simulink model "Quadcopter_LQR_Discrete"  (R2016b)
settings: Solver=ode45  StartTime=0.0  StopTime=50  RelTol=1e-3  EnableMultiTasking=on
undefined symbols (not defined in the file): C, F, sigbuilder_block, Ts, X0
settings Model: Creator=Toshiba  LastModifiedBy=AAstudillo
settings DataIOCC: LimitDataPoints=on  SaveFormat=Array  SignalLoggingSaveFormat=ModelDataLogs
settings OptimizationCC: LifeSpan=inf
settings DebuggingCC: SolverPrmCheckMsg=warning  MultiTaskDSMMsg=warning  MultiTaskCondExecSysMsg=none  SFUnexpectedBacktrackingDiag=warning  SFNoUnconditionalDefaultTransitionDiag=warning  SFExecutionAtInitializationDiag=none
settings HardwareCC: ProdBitPerPointer=32  ProdBitPerSizeT=32  ProdBitPerPtrDiffT=32  ProdLargestAtomicFloat=None  ProdIntDivRoundTo=Undefined  ProdEndianess=Unspecified  ProdWordSize=32  ProdHWDeviceType=32-bit Generic
settings ModelReferenceCC: PropagateSignalLabelsOutOfModel=off
settings GRTTargetCC: TargetLangStandard=C89/C90 (ANSI)  GeneratePreprocessorConditionals=Disable all
settings ConfigComp: CovMetricSettings=dw  CovHtmlReporting=on  CovSaveCumulativeToWorkspaceVar=on  CovSaveSingleToWorkspaceVar=on  CovExternalEMLEnable=off

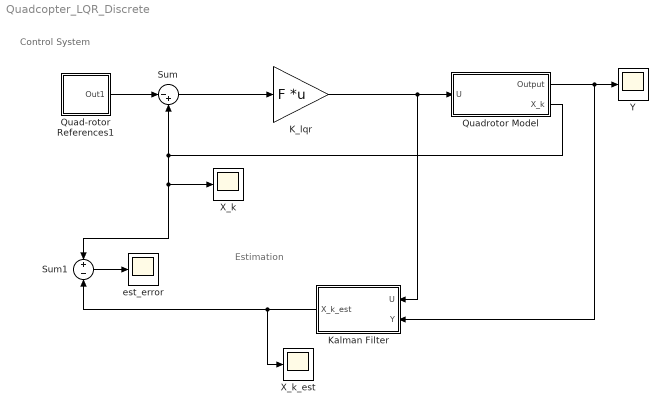
== system Quadcopter_LQR_Discrete ==
  note: Estimation
  note: Control System
  K_lqr : Gain  Gain=F  Multiplication=Matrix(K*u) (u vector)
  Kalman Filter : Subsystem
  Quad-rotor References1 : Subsystem
  Quadrotor Model : Subsystem
  Sum : Sum  Inputs=|-+
  Sum1 : Sum  Inputs=+|-
  X_k : Scope
  X_k_est : Scope
  Y : Scope
  est_error : Scope
  wires:
  K_lqr/1 -> Quadrotor Model/1(U), Kalman Filter/1(U)
  Sum/1 -> K_lqr/1
  Quadrotor Model/1("Output ") -> Y/1, Kalman Filter/2(Y)
  Quad-rotor References1/1(Out1) -> Sum/1
  Quadrotor Model/2(X_k) -> Sum1/1, X_k/1, Sum/2
  Kalman Filter/1("X_k_est ") -> X_k_est/1, Sum1/2
  Sum1/1 -> est_error/1

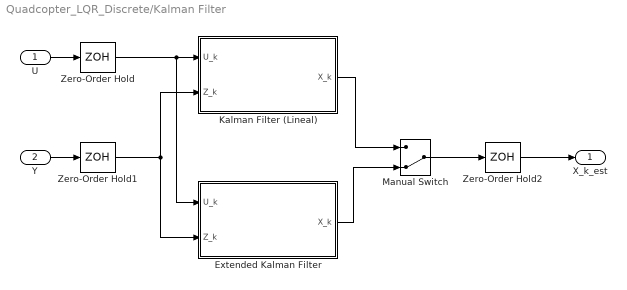
== system Quadcopter_LQR_Discrete/Kalman Filter ==
  U : Inport  PortDimensions=4
  Y : Inport  Port=2
  Extended Kalman Filter : MATLAB Function  TreatAsAtomicUnit=on
  Kalman Filter (Lineal) : MATLAB Function  TreatAsAtomicUnit=on
  Manual Switch : ManualSwitch  CurrentSetting=0
  Zero-Order Hold : ZeroOrderHold  SampleTime=Ts
  Zero-Order Hold1 : ZeroOrderHold  SampleTime=Ts
  Zero-Order Hold2 : ZeroOrderHold  SampleTime=Ts
  "X_k_est " : Outport  PortDimensions=12
  wires:
  U/1 -> Zero-Order Hold/1
  Zero-Order Hold/1 -> Extended Kalman Filter/1(U_k), Kalman Filter (Lineal)/1(U_k)
  Y/1 -> Zero-Order Hold1/1
  Zero-Order Hold1/1 -> Extended Kalman Filter/2(Z_k), Kalman Filter (Lineal)/2(Z_k)
  Kalman Filter (Lineal)/1(X_k) -> Manual Switch/1
  Zero-Order Hold2/1 -> "X_k_est "/1
  Extended Kalman Filter/1(X_k) -> Manual Switch/2
  Manual Switch/1 -> Zero-Order Hold2/1

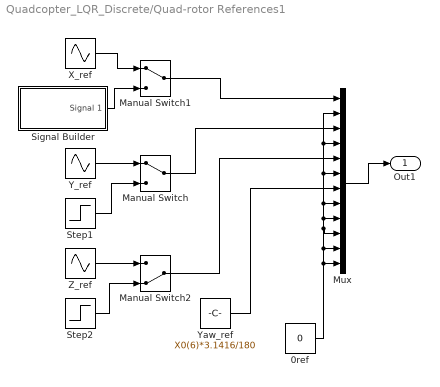
== system Quadcopter_LQR_Discrete/Quad-rotor References1 ==
  "0ref " : Constant  Value=0
  Manual Switch : ManualSwitch
  Manual Switch1 : ManualSwitch
  Manual Switch2 : ManualSwitch  CurrentSetting=0
  Mux : Mux  Inputs=12
  Signal Builder : Subsystem  Tag=STV Subsys  LoadFcn=sigbuilder_block('load');  StartFcn=sigbuilder_block('start');  StopFcn=sigbuilder_block('stop');  ClipboardFcn=sigbuilder_block('clipboard');  mask(Sigbuilder block){tuvar=[0:10]}
      mask help: Simulink:masks:SigbuilderBlock_MD
      mask init:
      | if ~strcmp(get_param(bdroot(gcbh),'SimulationStatus'),'stopped') tuvar = sigbuilder_block('maskInit'); end
      settings: CopyFcn=sigbuilder_block('copy');  DeleteFcn=sigbuilder_block('delete');  ModelCloseFcn=sigbuilder_block('modelClose');  PreSaveFcn=sigbuilder_block('preSave');  PauseFcn=sigbuilder_block('pause');  ContinueFcn=sigbuilder_block('continue');  NameChangeFcn=sigbuilder_block('namechange');  OpenFcn=sigbuilder_block('open',[6 30 1012.5 447.75 ]);  CloseFcn=sigbuilder_block('close');
      mask Display: plot(0, 0, 100, 100,[2, 2, 32, 32, 2], [68, 8, 8, 68, 68],[32, 2], [38, 38], [32, 19, 2],[53, 60, 44], [32, 17, 17, 2],[16, 16, 31, 31]);txt = getActiveGroup(gcbh);text(2, 100, txt,'verticalAlignment', 'top');
  Step1 : Step  Time=20  Before=1  After=0  SampleTime=0
  Step2 : Step  Time=20  Before=1  After=2  SampleTime=0
  X_ref : Sin  Frequency=3.141592654*0.025  SampleTime=0
  Y_ref : Sin  Frequency=3.141592654*0.025  Phase=3.141592654/2  SampleTime=0
  Yaw_ref : Constant  Value=X0(6)*3.1416/180
  Z_ref : Sin  Bias=1  Frequency=3.141592654*0.05  Phase=3.141592654  SampleTime=0
  Out1 : Outport
  wires:
  Mux/1 -> Out1/1
  X_ref/1 -> Manual Switch1/1
  Signal Builder/1(Signal 1) -> Manual Switch1/2
  Y_ref/1 -> Manual Switch/1
  Step1/1 -> Manual Switch/2
  Step2/1 -> Manual Switch2/2
  Z_ref/1 -> Manual Switch2/1
  Manual Switch1/1 -> Mux/1
  Manual Switch/1 -> Mux/3
  Manual Switch2/1 -> Mux/5
  Yaw_ref/1 -> Mux/7
  "0ref "/1 -> Mux/12, Mux/11, Mux/10, Mux/9, Mux/8, Mux/6, Mux/4, Mux/2

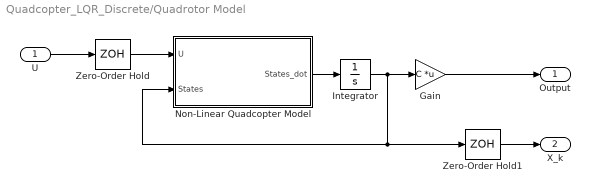
== system Quadcopter_LQR_Discrete/Quadrotor Model ==
  U : Inport
  Gain : Gain  Gain=C  Multiplication=Matrix(K*u)
  Integrator : Integrator  InitialCondition=X0
  Non-Linear Quadcopter Model : MATLAB Function  TreatAsAtomicUnit=on
  Zero-Order Hold : ZeroOrderHold  SampleTime=Ts
  Zero-Order Hold1 : ZeroOrderHold  SampleTime=Ts
  "Output " : Outport
  X_k : Outport  Port=2
  wires:
  Non-Linear Quadcopter Model/1(States_dot) -> Integrator/1
  Zero-Order Hold/1 -> Non-Linear Quadcopter Model/1(U)
  U/1 -> Zero-Order Hold/1
  Gain/1 -> "Output "/1
  Integrator/1 -> Gain/1, Non-Linear Quadcopter Model/2(States), Zero-Order Hold1/1
  Zero-Order Hold1/1 -> X_k/1

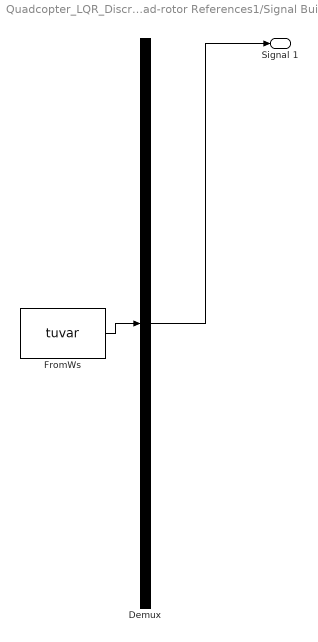
== system Quadcopter_LQR_Discrete/Quad-rotor References1/Signal Builder ==
  Demux : Demux  Tag=STV Demux  Outputs=1
  FromWs : FromWorkspace  Tag=STV FromWs  VariableName=tuvar  SampleTime=0
      SigBuilderData=|
      | common.afterFinalStr = 'Extrapolate'
      | common.sampleTime = 0
      | dataSet.timeRange = [0 30]
      | dataSet.name = 'Group 1'
      | sbobj.Groups.Name = 'Group 1'
      | sbobj.Groups.Signals.Name = 'Signal 1'
      | sbobj.Groups.Signals.XData = [0 4 5 6 10 10 30]
      | sbobj.Groups.Signals.YData = [0 0 0.14 0.48 0.925 0.99 0.99]
      | sbobj.Groups.TimeRange = [0 30]
  Signal 1 : Outport  Tag=STV Outport
  wires:
  Demux/1 -> Signal 1/1
  FromWs/1 -> Demux/1

== matlab function Quadcopter_LQR_Discrete/Kalman Filter/Extended Kalman Filter ==
  data: U_k input; Z_k input; X_k output
function X_k  = fcn(U_k, Z_k)

    % Declare two persistent variables 'X_k_1' and 'P_k_1'.
    persistent X_k_1 P_k_1;

    % Upon the first call we need to initialize the variables.
    if isempty(X_k_1)
        X_k_1 = zeros(12,1); % This can be modified
    end
    if isempty(P_k_1)
        P_k_1 = 100*eye(12); % This can be modified
    end
    
    A_k = [
         1    0.0100         0         0         0         0         0         0    0.0005    0.0000         0         0;
         0    1.0000         0         0         0         0         0         0    0.0981    0.0005         0         0;
         0         0    1.0000    0.0100         0         0         0         0         0         0    0.0005    0.0000;
         0         0         0    1.0000         0         0         0         0         0         0    0.0981    0.0005;
         0         0         0         0    1.0000    0.0100         0         0         0         0         0         0;
         0         0         0         0         0    1.0000         0         0         0         0         0         0;
         0         0         0         0         0         0    1.0000    0.0100         0         0         0         0;
         0         0         0         0         0         0         0    1.0000         0         0         0         0;
         0         0         0         0         0         0         0         0    1.0000    0.0100         0         0;
         0         0         0         0         0         0         0         0         0    1.0000         0         0;
         0         0         0         0         0         0         0         0         0         0    1.0000    0.0100;
         0         0         0         0         0         0         0         0         0         0         0    1.0000];
    B_k = [0         0    0.0000         0;
           0         0    0.0001         0;
           0         0         0    0.0000;
           0         0         0    0.0001;
      0.0000         0         0         0;
      0.0064         0         0         0;
           0    0.0015         0         0;
           0    0.2976         0         0;
           0         0    0.0040         0;
           0         0    0.8064         0;
           0         0         0    0.0037;
           0         0         0    0.7407];
       
    Q_kf = 0.001*eye(12); % THIS MUST BE MODIFIED
    R_kf = 3*eye(4);  % THIS MUST BE MODIFIED
    
    H = [1 0 0 0 0 0 0 0 0 0 0 0;
         0 0 1 0 0 0 0 0 0 0 0 0;
         0 0 0 0 1 0 0 0 0 0 0 0;
         0 0 0 0 0 0 1 0 0 0 0 0];

    %Predict
    Xk_ = A_k*X_k_1 + B_k*U_k;
    Pk_ = A_k*P_k_1*A_k' + Q_kf;

    %Optimal Kalman gain
    K_k = Pk_*H'/(H*Pk_*H'+R_kf);

    %Update            
    X_k = Xk_ + K_k*(Z_k - H*(Xk_));
    P_k = (eye(12)-K_k*H)*Pk_;

    %Modified the persitent variables
    X_k_1 = X_k;
    P_k_1 = P_k;

== matlab function Quadcopter_LQR_Discrete/Quadrotor Model/Non-Linear Quadcopter Model ==
  data: U input; States input; States_dot output
function States_dot  = fcn(U, States)

% Gravity constant
              g = 9.807;

              m = 1.568;
              Ixx = 0.0135;
              Iyy = 0.0124;
              Izz = 0.0336;

    %Inputs = U, States
    %Outputs = States_dot  
    %States: X dX Y dY Z dZ Psi dPsi Theta dTheta Phi dPhi
    %        1  2 3  4 5  6  7   8     9      10   11  12
    
    U1 = U(1)+m*g;
    U2 = U(2);
    U3 = U(3);
    U4 = U(4);

    dX = States(2);
    ddX = (U1/m)*(cos(States(7))*sin(States(9))*cos(States(11)) + sin(States(7))*sin(States(11)));
    %ddX = -States(10)*States(6) + States(8)*States(4) + g*sin(States(9));
    dY = States(4);
    ddY = (U1/m)*(-sin(States(7))*sin(States(9))*cos(States(11)) + cos(States(7))*sin(States(11)));
    %ddY = States(8)*States(2) - States(12)*States(6) + g*cos(States(9))*sin(States(11));
    dZ = States(6);
    ddZ = ((U1/m)*cos(States(9))*cos(States(11))) - g;
    %ddZ = States(10)*States(2) - States(12)*States(4) - g*cos(States(9))*cos(States(11)) + (U1)/m;
    
    dPsi = States(8);
    ddPsi = (((Ixx-Iyy)/Izz)*States(12)*States(10)) + (U2/Izz);
    dTheta = States(10);
    ddTheta = (((Izz-Ixx)/Iyy)*States(12)*States(8)) + (U3/Iyy);
    dPhi = States(12);
    ddPhi = (((Iyy-Izz)/Ixx)*States(10)*States(8)) + (U4/Ixx);

States_dot = [dX, ddX, dY, ddY, dZ, ddZ, dPsi, ddPsi, dTheta, ddTheta, dPhi, ddPhi]';

== matlab function Quadcopter_LQR_Discrete/Kalman Filter/Kalman Filter (Lineal) ==
  data: U_k input; Z_k input; X_k output
function X_k  = fcn(U_k, Z_k)

    % Declare two persistent variables 'X_k_1' and 'P_k_1'.
    persistent X_k_1 P_k_1;

    % Upon the first call we need to initialize the variables.
    if isempty(X_k_1)
        X_k_1 = zeros(12,1); % This can be modified
    end
    if isempty(P_k_1)
        P_k_1 = 100*eye(12); % This can be modified
    end
    
    A_k = [
         1    0.0100         0         0         0         0         0         0    0.0005    0.0000         0         0;
         0    1.0000         0         0         0         0         0         0    0.0981    0.0005         0         0;
         0         0    1.0000    0.0100         0         0         0         0         0         0    0.0005    0.0000;
         0         0         0    1.0000         0         0         0         0         0         0    0.0981    0.0005;
         0         0         0         0    1.0000    0.0100         0         0         0         0         0         0;
         0         0         0         0         0    1.0000         0         0         0         0         0         0;
         0         0         0         0         0         0    1.0000    0.0100         0         0         0         0;
         0         0         0         0         0         0         0    1.0000         0         0         0         0;
         0         0         0         0         0         0         0         0    1.0000    0.0100         0         0;
         0         0         0         0         0         0         0         0         0    1.0000         0         0;
         0         0         0         0         0         0         0         0         0         0    1.0000    0.0100;
         0         0         0         0         0         0         0         0         0         0         0    1.0000];
    B_k = [0         0    0.0000         0;
           0         0    0.0001         0;
           0         0         0    0.0000;
           0         0         0    0.0001;
      0.0000         0         0         0;
      0.0064         0         0         0;
           0    0.0015         0         0;
           0    0.2976         0         0;
           0         0    0.0040         0;
           0         0    0.8064         0;
           0         0         0    0.0037;
           0         0         0    0.7407];
       
    Q_kf = 0.001*eye(12); % THIS MUST BE MODIFIED
    R_kf = 3*eye(4);  % THIS MUST BE MODIFIED
    
    H = [1 0 0 0 0 0 0 0 0 0 0 0;
         0 0 1 0 0 0 0 0 0 0 0 0;
         0 0 0 0 1 0 0 0 0 0 0 0;
         0 0 0 0 0 0 1 0 0 0 0 0];

    %Predict
    Xk_ = A_k*X_k_1 + B_k*U_k;
    Pk_ = A_k*P_k_1*A_k' + Q_kf;

    %Optimal Kalman gain
    K_k = Pk_*H'/(H*Pk_*H'+R_kf);

    %Update            
    X_k = Xk_ + K_k*(Z_k - H*(Xk_));
    P_k = (eye(12)-K_k*H)*Pk_;

    %Modified the persitent variables
    X_k_1 = X_k;
    P_k_1 = P_k;
